simulink model "TestRotation"  (R2022a)
settings: Solver=VariableStepAuto  StartTime=0.0  StopTime=10.0  RelTol=1e-3
undefined symbols (not defined in the file): axleLength, InputPWM, ticksPerRot, wheelR, WheelSpeed
libraries: arduinolib x8, spsEdgeDetectorLib x2, simulink x1, slpidlib x1, mobileRoboticsTrainingLib x1
settings Model: Creator=ryanj  LastModifiedBy=ryanj

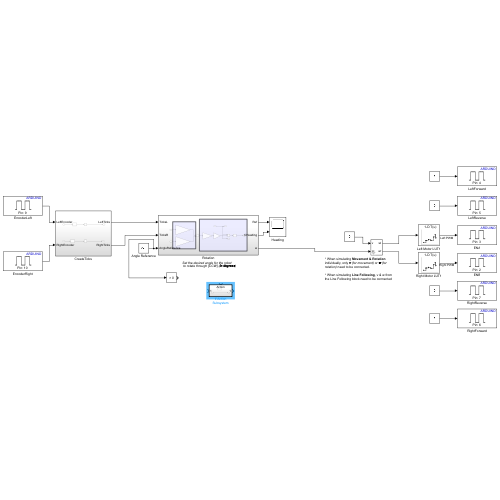
[thumbnail: Simulink's stored preview of the top-level diagram]
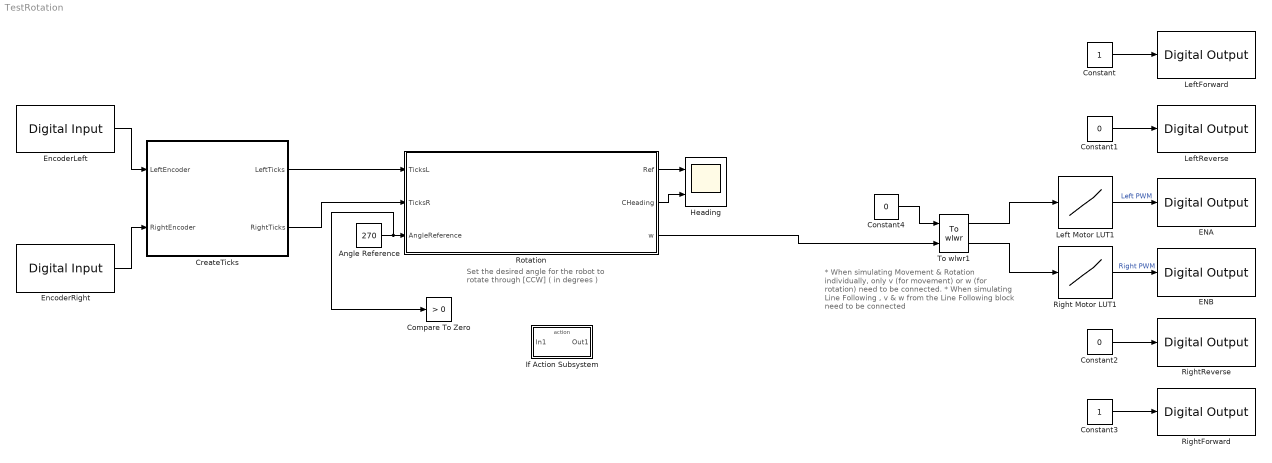
== system TestRotation ==
  note: * When simulating Movement & Rotation individually, only v (for movement) or w (for rotation) need to be connected.
      |
      | * When simulating Line Following , v & w from the Line Following block need to be connected
  note: Set the desired angle for the robot
      | to rotate through [CCW] ( in degrees )
  Angle Reference : Constant  Value=270
  Compare To Zero : simulink/Logic and Bit Operations/Compare To Zero  relop=>  OutDataTypeStr=boolean
  Constant : Constant
  Constant1 : Constant  Value=0
  Constant2 : Constant  Value=0
  Constant3 : Constant
  Constant4 : Constant  Value=0
  CreateTicks : Subsystem
  ENA : arduinolib/Digital Output  pinNumber=3  Direction=output  blockPlatform=arduino
  ENB : arduinolib/Digital Output  pinNumber=2  Direction=output  blockPlatform=arduino
  EncoderLeft : arduinolib/Digital Input  pinNumber=9  mode=Default  Direction=input  SampleTime=0.1  blockPlatform=arduino
  EncoderRight : arduinolib/Digital Input  pinNumber=10  mode=Default  Direction=input  SampleTime=0.1  blockPlatform=arduino
  Heading : Scope  NumInputPorts=2
  If Action Subsystem : Subsystem  TreatAsAtomicUnit=on
  Left Motor LUT1 : Lookup_n-D  NumberOfTableDimensions=1  BreakpointsForDimension1=WheelSpeed  Table=InputPWM  InterpMethod=Nearest  ExtrapMethod=Clip  InternalRulePriority=Speed  RndMeth=Simplest
  LeftForward : arduinolib/Digital Output  pinNumber=4  Direction=output  blockPlatform=arduino
  LeftReverse : arduinolib/Digital Output  pinNumber=5  Direction=output  blockPlatform=arduino
  Right Motor LUT1 : Lookup_n-D  NumberOfTableDimensions=1  BreakpointsForDimension1=WheelSpeed  Table=InputPWM  InterpMethod=Nearest  ExtrapMethod=Clip  InternalRulePriority=Speed  RndMeth=Simplest
  RightForward : arduinolib/Digital Output  pinNumber=6  Direction=output  blockPlatform=arduino
  RightReverse : arduinolib/Digital Output  pinNumber=7  Direction=output  blockPlatform=arduino
  Rotation : Subsystem
  To wlwr1 : mobileRoboticsTrainingLib/To wlwr  axleLength=0.1  wheelR=0.05
  wires:
  Right Motor LUT1/1 -> ENB/1  "Right PWM"
  To wlwr1/1 -> Left Motor LUT1/1
  To wlwr1/2 -> Right Motor LUT1/1
  Left Motor LUT1/1 -> ENA/1  "Left PWM"
  Constant/1 -> LeftForward/1
  Constant3/1 -> RightForward/1
  EncoderRight/1 -> CreateTicks/2(RightEncoder)
  Constant1/1 -> LeftReverse/1
  Constant2/1 -> RightReverse/1
  EncoderLeft/1 -> CreateTicks/1(LeftEncoder)
  Rotation/2(CHeading) -> Heading/2
  Angle Reference/1 -> Compare To Zero/1, Rotation/3(AngleReference)
  Rotation/1(Ref) -> Heading/1
  CreateTicks/1(LeftTicks) -> Rotation/1(TicksL)
  CreateTicks/2(RightTicks) -> Rotation/2(TicksR)
  Rotation/3(w) -> To wlwr1/2
  Constant4/1 -> To wlwr1/1

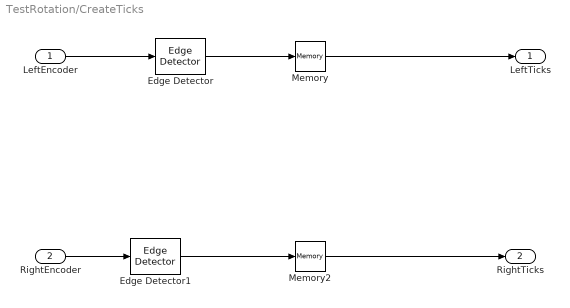
== system TestRotation/CreateTicks ==
  LeftEncoder : Inport
  RightEncoder : Inport  Port=2
  Edge Detector : spsEdgeDetectorLib/Edge Detector  model=Rising  ic=0  Ts=0
      settings: SourceProductBaseCode=PS
  Edge Detector1 : spsEdgeDetectorLib/Edge Detector  model=Rising  ic=0  Ts=0
      settings: SourceProductBaseCode=PS
  Memory : Memory
  Memory2 : Memory
  LeftTicks : Outport
  RightTicks : Outport  Port=2
  wires:
  Memory/1 -> LeftTicks/1
  RightEncoder/1 -> Edge Detector1/1
  LeftEncoder/1 -> Edge Detector/1
  Edge Detector/1 -> Memory/1
  Edge Detector1/1 -> Memory2/1
  Memory2/1 -> RightTicks/1

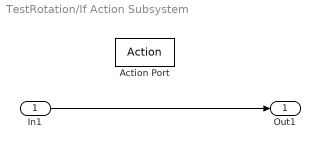
== system TestRotation/If Action Subsystem ==
  In1 : Inport
  Action Port : ActionPort
  Out1 : Outport
  wires:
  In1/1 -> Out1/1

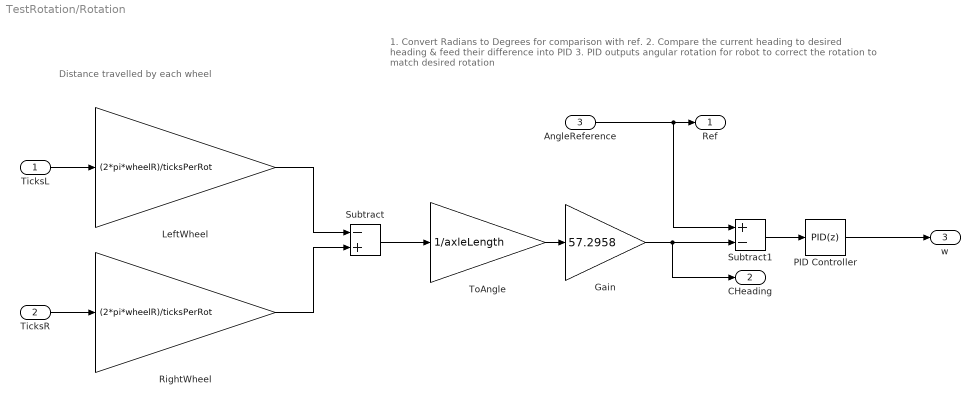
== system TestRotation/Rotation ==
  note: 1. Convert Radians to Degrees for comparison with ref.
      | 2. Compare the current heading to desired heading
      | & feed their difference into PID
      | 3. PID outputs angular rotation for robot to correct
      | the rotation to match desired rotation
  note: Distance travelled by each wheel
  TicksL : Inport
  TicksR : Inport  Port=2
  AngleReference : Inport  Port=3
  Gain : Gain  Gain=57.2958
  LeftWheel : Gain  Gain=(2*pi*wheelR)/ticksPerRot
  PID Controller : slpidlib/PID Controller  Controller=PID  Form=Parallel  TimeDomain=Discrete-time  UseExternalTs=off  SampleTime=-1  IntegratorMethod=Forward Euler  FilterMethod=Forward Euler  ControllerParametersSource=internal  P=0.111  I=0.001  UseKiTs=off  D=0  N=100  UseFilter=off  TunerSelectOption=Transfer Function Based (PID Tuner App)  InitialConditionSource=internal  InitialConditionForIntegrator=0  InitialConditionForFilter=0  DifferentiatorICPrevScaledInput=0  ExternalReset=none  TrackingMode=off  Kt=1  LimitOutput=on  SatLimitsSource=internal  UpperSaturationLimit=4  LowerSaturationLimit=-4  LinearizeAsGain=on  AntiWindupMode=clamping  Kb=1  POutMin=[]  POutMax=[]  IOutMin=[]  IOutMax=[]  DOutMin=[]  DOutMax=[]  NOutMin=[]  NOutMax=[]  SumOutMin=[]  SumOutMax=[]  SaturationOutMin=[]  SaturationOutMax=[]  PParamMin=[]  PParamMax=[]  IParamMin=[]  IParamMax=[]  DParamMin=[]  DParamMax=[]  NParamMin=[]  NParamMax=[]  KbParamMin=[]  KbParamMax=[]  KtParamMin=[]  KtParamMax=[]  KbOutMin=[]  KbOutMax=[]  KtOutMin=[]  KtOutMax=[]  IntegratorOutMin=[]  IntegratorOutMax=[]  FilterOutMin=[]  FilterOutMax=[]  SumI1OutMin=[]  SumI1OutMax=[]  SumI2OutMin=[]  SumI2OutMax=[]  SumI3OutMin=[]  SumI3OutMax=[]  SumI4OutMin=[]  SumI4OutMax=[]  SumDOutMin=[]  SumDOutMax=[]  DifferentiatorOutMin=[]  DifferentiatorOutMax=[]  FilterDiffOutCoefMin=[]  FilterDiffOutCoefMax=[]  ReciprocalOutMin=[]  ReciprocalOutMax=[]  SumDenOutMin=[]  SumDenOutMax=[]  SumNumOutMin=[]  SumNumOutMax=[]  DivideOutMin=[]  DivideOutMax=[]  UdiffTsProdOutMin=[]  UdiffTsProdOutMax=[]  NTsProdOutMin=[]  NTsProdOutMax=[]  UintegralTsProdOutMin=[]  UintegralTsProdOutMax=[]  UngainTsProdOutMin=[]  UngainTsProdOutMax=[]  IntegratorContinuousStateAttributes=''  IntegratorStateMustResolveToSignalObject=off  IntegratorRTWStateStorageClass=Auto  FilterContinuousStateAttributes=''  FilterStateMustResolveToSignalObject=off  FilterRTWStateStorageClass=Auto  ParallelPVariant=InternalParameters  IdealPVariant=Disabled  IVariant=InternalParameters  DVariant=InternalParameters  IntegratorVariant=Discrete  SatVariant=Enabled  AWVariant=DiscClampingParallel  PCopyVariant=Disabled  TRVariant=Disabled  FdbkBlocksVariant=Forward  IdealPFdbkVariant=Disabled  SatFdbkVariant=Disabled  DerivativeFilterVariant=Differentiator  NVariant=Passthrough  NCopyVariant=Disabled_SignalSpec  FilterICVariant=InternalICsDifferentiator  IntegratorICVariant=InternalICs  ExternalResetVariant=Disabled  TRSumVariant=Passthrough  SumFdbkVariant=Disabled  SumVariant=Sum_PID  TsampFilterVariant=InternalTs  TsampNgainVariant=Passthrough  TsampIntegralVariant=Passthrough  ExternalSaturationOutDataTypeStr=Inherit: Same as second input  aMode=0  InitialConditionSetting=Output
  RightWheel : Gain  Gain=(2*pi*wheelR)/ticksPerRot
  Subtract : Sum  Inputs=-+
  Subtract1 : Sum  Inputs=+-
  ToAngle : Gain  Gain=1/axleLength
  Ref : Outport
  CHeading : Outport  Port=2
  w : Outport  Port=3
  wires:
  RightWheel/1 -> Subtract/2
  LeftWheel/1 -> Subtract/1
  Subtract/1 -> ToAngle/1
  Subtract1/1 -> PID Controller/1
  Gain/1 -> CHeading/1, Subtract1/2
  AngleReference/1 -> Ref/1, Subtract1/1
  TicksL/1 -> LeftWheel/1
  ToAngle/1 -> Gain/1
  TicksR/1 -> RightWheel/1
  PID Controller/1 -> w/1
